simulink model "bloculfiltru"  (R2023b)
settings: Solver=VariableStepAuto  StartTime=0.0  StopTime=10.0  RelTol=1e-3
settings Model: Creator=diana.forrai  LastModifiedBy=diana.forrai

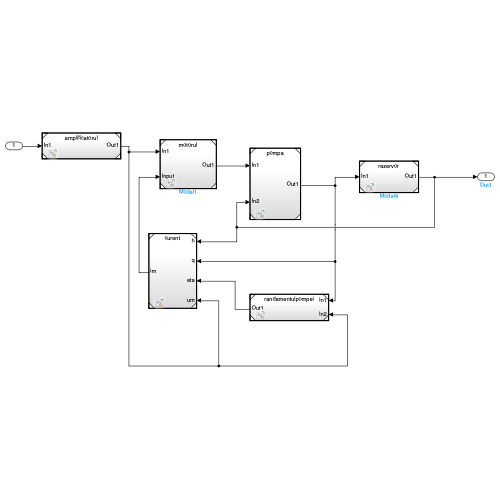
[thumbnail: Simulink's stored preview of the top-level diagram]
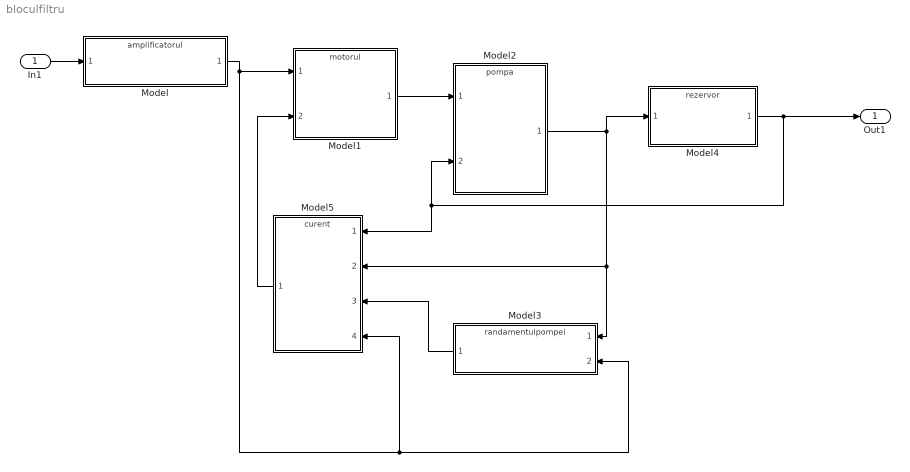
== system bloculfiltru ==
  In1 : Inport
  Model : ModelReference  ModelNameDialog=amplificatorul.slx  SimulationMode=Normal  ModelReferenceVersion=1.1
  Model1 : ModelReference  ModelNameDialog=motorul.slx  SimulationMode=Normal  ModelReferenceVersion=1.1
  Model2 : ModelReference  ModelNameDialog=pompa.slx  SimulationMode=Normal  ModelReferenceVersion=1.1
  Model3 : ModelReference  ModelNameDialog=randamentulpompei.slx  SimulationMode=Normal  ModelReferenceVersion=1.2
  Model4 : ModelReference  ModelNameDialog=rezervor.slx  SimulationMode=Normal  ModelReferenceVersion=1.2
  Model5 : ModelReference  ModelNameDialog=curent.slx  SimulationMode=Normal  ModelReferenceVersion=1.1
  Out1 : Outport
  wires:
  In1/1 -> Model/1
  Model1/1 -> Model2/1
  Model2/1 -> Model4/1, Model5/2, Model3/1
  Model3/1 -> Model5/3
  Model5/1 -> Model1/2
  Model/1 -> Model5/4, Model3/2, Model1/1
  Model4/1 -> Model5/1, Model2/2, Out1/1
